simulink model "wipr_crtl_sys_mdl"  (R2024b)
settings: Solver=FixedStepDiscrete  StartTime=0.0  StopTime=10.0  FixedStep=0.01  RelTol=1e-3
settings Model: Creator=Hassan Mohamed  LastModifiedBy=Hassan Mohamed

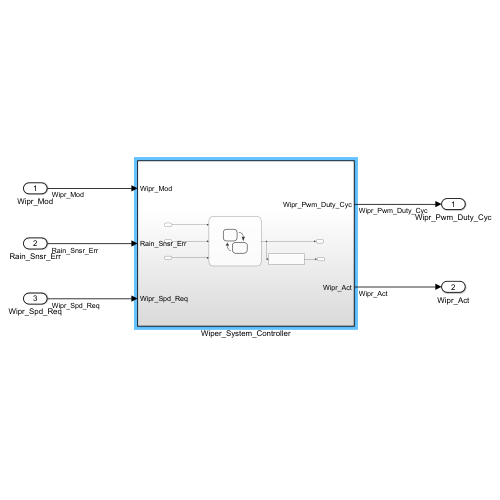
[thumbnail: Simulink's stored preview of the top-level diagram]
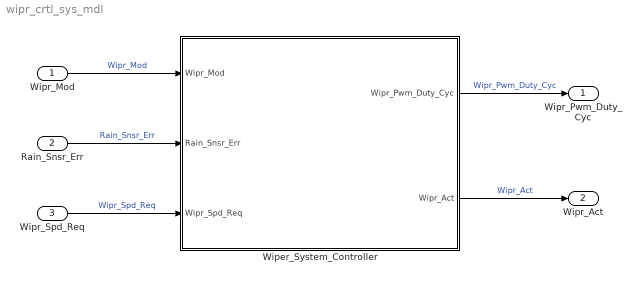
== system wipr_crtl_sys_mdl ==
  Wipr_Mod : Inport  OutMin=0  OutMax=3  OutDataTypeStr=uint8
  Rain_Snsr_Err : Inport  Port=2  OutMin=0  OutMax=1  OutDataTypeStr=boolean
  Wipr_Spd_Req : Inport  Port=3  OutMin=0  OutMax=7  OutDataTypeStr=uint8
  Wiper_System_Controller : Subsystem
  Wipr_Pwm_Duty_Cyc : Outport  OutMin=0  OutMax=1  OutDataTypeStr=single
  Wipr_Act : Outport  Port=2  OutMin=0  OutMax=1  OutDataTypeStr=boolean
  wires:
  Wipr_Spd_Req/1 -> Wiper_System_Controller/3(Wipr_Spd_Req)  "Wipr_Spd_Req"
  Rain_Snsr_Err/1 -> Wiper_System_Controller/2(Rain_Snsr_Err)  "Rain_Snsr_Err"
  Wipr_Mod/1 -> Wiper_System_Controller/1(Wipr_Mod)  "Wipr_Mod"
  Wiper_System_Controller/1(Wipr_Pwm_Duty_Cyc) -> Wipr_Pwm_Duty_Cyc/1  "Wipr_Pwm_Duty_Cyc"
  Wiper_System_Controller/2(Wipr_Act) -> Wipr_Act/1  "Wipr_Act"

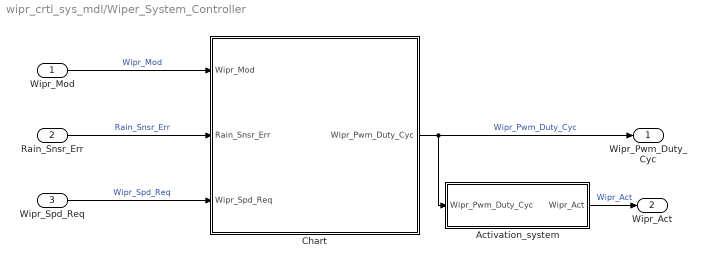
== system wipr_crtl_sys_mdl/Wiper_System_Controller ==
  Wipr_Mod : Inport  OutMin=0  OutMax=3  OutDataTypeStr=uint8
  Rain_Snsr_Err : Inport  Port=2  OutMin=0  OutMax=1  OutDataTypeStr=boolean
  Wipr_Spd_Req : Inport  Port=3  OutDataTypeStr=uint8
  Activation_system : Subsystem
  Chart : Stateflow chart  TreatAsAtomicUnit=on
  Wipr_Pwm_Duty_Cyc : Outport  OutMin=0  OutMax=1  OutDataTypeStr=single
  Wipr_Act : Outport  Port=2  OutMin=0  OutMax=1  OutDataTypeStr=boolean
  wires:
  Wipr_Mod/1 -> Chart/1(Wipr_Mod)  "Wipr_Mod"
  Rain_Snsr_Err/1 -> Chart/2(Rain_Snsr_Err)  "Rain_Snsr_Err"
  Chart/1(Wipr_Pwm_Duty_Cyc) -> Activation_system/1(Wipr_Pwm_Duty_Cyc), Wipr_Pwm_Duty_Cyc/1  "Wipr_Pwm_Duty_Cyc"
  Wipr_Spd_Req/1 -> Chart/3(Wipr_Spd_Req)  "Wipr_Spd_Req"
  Activation_system/1(Wipr_Act) -> Wipr_Act/1  "Wipr_Act"

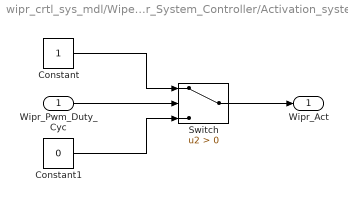
== system wipr_crtl_sys_mdl/Wiper_System_Controller/Activation_system ==
  Wipr_Pwm_Duty_Cyc : Inport  OutDataTypeStr=single
  Constant : Constant  OutDataTypeStr=boolean
  Constant1 : Constant  Value=0  OutDataTypeStr=boolean
  Switch : Switch  Criteria=u2 > Threshold  SaturateOnIntegerOverflow=off  InputSameDT=off
  Wipr_Act : Outport  OutDataTypeStr=boolean
  wires:
  Wipr_Pwm_Duty_Cyc/1 -> Switch/2
  Switch/1 -> Wipr_Act/1
  Constant/1 -> Switch/1
  Constant1/1 -> Switch/3

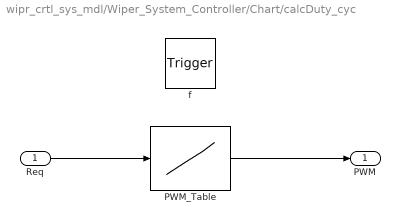
== system wipr_crtl_sys_mdl/Wiper_System_Controller/Chart/calcDuty_cyc ==
  Req : Inport  OutDataTypeStr=uint8  PortDimensions=1
  f : TriggerPort  TriggerType=function-call  VariantControl=(inherit)
      settings: CopyFcn=Stateflow.SLINSF.SimulinkMan.removeBlockPreDeleteFcn  PreDeleteFcn=Stateflow.SLINSF.SimulinkMan.unsafePredeleteFcn
  PWM_Table : Lookup_n-D  NumberOfTableDimensions=1  BreakpointsForDimension1=[0 1 2 3 4 5 6 7]  Table=[0 0.4 0.45 0.5 0.55 0.6 0.65 0.7]  ExtrapMethod=Clip  InternalRulePriority=Speed  OutDataTypeStr=single  RndMeth=Simplest
  PWM : Outport  OutMin=0  OutMax=1  OutDataTypeStr=single
  wires:
  Req/1 -> PWM_Table/1
  PWM_Table/1 -> PWM/1

== stateflow chart wipr_crtl_sys_mdl/Wiper_System_Controller/Chart ==
  state PWM = calcDuty_cyc( Req) [function]
  state Off
    en:
    Wipr_Pwm_Duty_Cyc = 0;
    du:
    Wipr_Pwm_Duty_Cyc = 0;
  state Auto_Mode
    en:
    Wipr_Pwm_Duty_Cyc = calcDuty_cyc(Wipr_Spd_Req);
    du:
    Wipr_Pwm_Duty_Cyc = calcDuty_cyc(Wipr_Spd_Req);
  state Low_Speed
    en:
    Wipr_Pwm_Duty_Cyc = 0.4;
    du:
    Wipr_Pwm_Duty_Cyc = 0.4;
  state High_Speed
    en:
    Wipr_Pwm_Duty_Cyc = 0.7;
    du:
    Wipr_Pwm_Duty_Cyc = 0.7;
  (default) -> Off
  Off -> (junction 11) : [Wipr_Mod ~= 0 && Rain_Snsr_Err==false]
  Auto_Mode -> (junction 11) : [Wipr_Mod ~= 1 || Rain_Snsr_Err == true]
  (junction 11) -> (junction 13)
  (junction 14) -> Off [order 1] : [Wipr_Mod == 0 || ...
      | (Wipr_Mod == 1 && Rain_Snsr_Err == true)]
  (junction 15) -> Auto_Mode [order 1] : [Wipr_Mod == 1 && Rain_Snsr_Err == false]
  (junction 13) -> (junction 14) [order 1]
  (junction 13) -> (junction 15) [order 2]
  (junction 14) -> Low_Speed [order 2] : [Wipr_Mod == 2]
  (junction 12) -> (junction 13)
  (junction 15) -> High_Speed [order 2] : [Wipr_Mod == 3]
  Low_Speed -> (junction 12) : [Wipr_Mod ~= 2]
  High_Speed -> (junction 12) : [Wipr_Mod ~= 3]
  data: Req function_input uint8 size=1; PWM function_output single; Wipr_Mod input uint8; Rain_Snsr_Err input boolean; Wipr_Spd_Req input uint8; Wipr_Pwm_Duty_Cyc output single
